simulink model "EPS_sim_test_v5_R19a"  (R2018b)
settings: Solver=FixedStepAuto  StartTime=0.0  StopTime=tsimulation  FixedStep=delta_t  MaxStep=10  RelTol=1e-3
values from neighbouring files (symbols this model uses):
  C = Cbat*Nbp*3600    (= 37440)    [demoEPS.m]    (also in demoEPS_R2019a.m; demoEPS_v1.m; demoEPS_v1a.m; demoEPS_v1test.m)
  DOD_0 = 0    [demoEPS.m]    (also in demoEPS_R2019a.m; demoEPS_v1.m; demoEPS_v1a.m; demoEPS_v1test.m)
  eff_ADC1 = 0.6    [demoEPS_v5.m]
  eff_GPS = 0.94    [demoEPS_v5.m]
  eff_MTQ = 0.91    [demoEPS_v5.m]
  eff_OBC = 0.95    [demoEPS_v4.m]    (also in demoEPS_v5.m = 0.94)
  eff_RWA = 0.3    [demoEPS_v5.m]
  eff_S = 0.98    [demoEPS_v5.m]
  eff_UHF = 0.94    [demoEPS_v5.m]
  EN_ADCS1 = 1    [demoEPS_v5.m]
  EN_GPS = 1    [demoEPS_v5.m]
  EN_heat = 0    [demoEPS_v5.m]
  EN_MTQ = 1    [demoEPS_v5.m]
  EN_OBC = 1    [demoEPS_v5.m]
  EN_RWA = 1    [demoEPS_v5.m]
  EN_S = 1    [demoEPS_v5.m]
  EN_UHF = 1    [demoEPS_v5.m]
  I_BC_max = -input (4)    [battchargedischarge.m]    (also in demoEPS.m = 3; demoEPS_R2019a.m = 3; demoEPS_v1.m = 3; demoEPS_v1a.m = 3)
  I_BD_max = input (3)    [battchargedischarge.m]    (also in demoEPS.m = 5; demoEPS_R2019a.m = 5; demoEPS_v1.m = 5; demoEPS_v1a.m = 5)
  Nbs = math.ceil(Vbusmin/Vbatmin)    [calc_mass_EPS.m]    (also in demoEPS.m = 4; demoEPS_R2019a.m = 4; demoEPS_v1.m = 4; demoEPS_v1a.m = 4)
  P_ADC = 0.55    [demoEPS_v5.m]
  P_eps = 0.6    [demoEPS.m]    (also in demoEPS_R2019a.m; demoEPS_v1.m; demoEPS_v1a.m; demoEPS_v1test.m)
  P_GPS = 0.225    [demoEPS_v5.m]
  P_heater = 3    [demoEPS_v4.m]    (also in demoEPS_v5.m = 6)
  P_MTQ = 1.2    [demoEPS_v5.m]
  P_OBC = 2.15    [demoEPS_v5.m]
  P_RWA = 0.6    [demoEPS_v5.m]
  Psa = 48    [demoEPS.m]    (also in demoEPS_R2019a.m; demoEPS_v1.m; demoEPS_v1a.m; demoEPS_v1test.m)
  Torb = 2*pi*sqrt(a^3/(3.986004418E5))    [demoEPS_v4.m]    (also in demoEPS_v5.m)
libraries: simulink x3
settings Model: Creator=Ricardo  LastModifiedBy=colpari
settings DataIOCC: ReturnWorkspaceOutputs=on

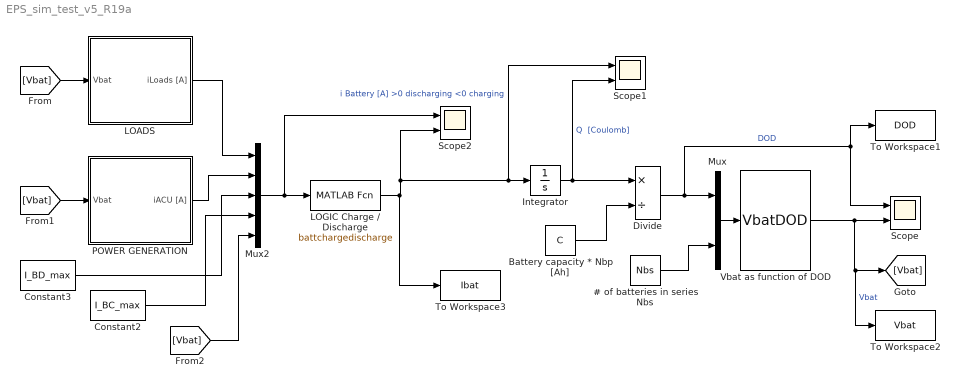
== system EPS_sim_test_v5_R19a ==
  # of batteries in series Nbs : Constant  Value=Nbs
  Battery capacity * Nbp [Ah] : Constant  Value=C
  Constant2 : Constant  Value=I_BC_max
  Constant3 : Constant  Value=I_BD_max
  Divide : Product  Inputs=*/
  Integrator : Integrator  InitialCondition=DOD_0
  LOADS : Subsystem
  LOGIC Charge / Discharge : MATLABFcn  MATLABFcn=battchargedischarge
  Mux : Mux  Inputs=2
  Mux2 : Mux  Inputs=5
  POWER GENERATION : Subsystem
  Scope : Scope  NumInputPorts=2
  Scope1 : Scope  NumInputPorts=2
  Scope2 : Scope  NumInputPorts=2
  To Workspace1 : ToWorkspace  VariableName=DOD  SaveFormat=Timeseries  SampleTime=-1
  To Workspace2 : ToWorkspace  VariableName=Vbat  SaveFormat=Timeseries  SampleTime=-1
  To Workspace3 : ToWorkspace  VariableName=Ibat  SaveFormat=Timeseries  SampleTime=-1
  Vbat as function of DOD : MATLABFcn  MATLABFcn=VbatDOD
  wires:
  Mux/1 -> Vbat as function of DOD/1
  # of batteries in series Nbs/1 -> Mux/2
  Vbat as function of DOD/1 -> To Workspace2/1, [Vbat], Scope/2  "Vbat"
  Divide/1 -> To Workspace1/1, Scope/1, Mux/1  "DOD"
  Integrator/1 -> Scope1/2, Divide/1  "Q  [Coulomb]"
  Battery capacity * Nbp [Ah]/1 -> Divide/2
  [Vbat] -> LOADS/1(Vbat)
  POWER GENERATION/1(iACU [A]) -> Mux2/2
  [Vbat] -> POWER GENERATION/1(Vbat)
  LOADS/1(iLoads [A]) -> Mux2/1
  Mux2/1 -> LOGIC Charge / Discharge/1, Scope2/1
  Constant3/1 -> Mux2/3
  Constant2/1 -> Mux2/4
  LOGIC Charge / Discharge/1 -> To Workspace3/1, Scope1/1, Integrator/1, Scope2/2  "i Battery [A] >0 discharging <0 charging"
  [Vbat] -> Mux2/5

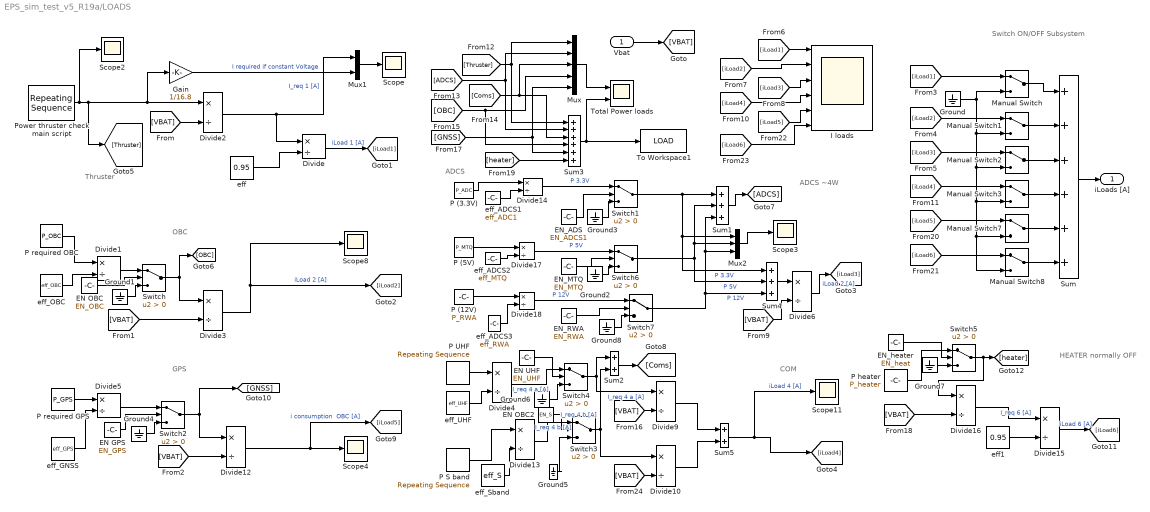
== system EPS_sim_test_v5_R19a/LOADS ==
  note: Switch
      | ON/OFF
      | Subsystem
  note: ADCS
  note: Thruster
  note: OBC
  note: ADCS ~4W
  note: COM
  note: GPS
  note: HEATER
      | normally
      | OFF
  Vbat : Inport
  Divide{,1..6,9..10,12..18} (16 alike) : Product  Inputs=*/
  EN GPS : Constant  Value=EN_GPS
  EN OBC : Constant  Value=EN_OBC
  EN OBC2 : Constant  Value=EN_S
  EN UHF : Constant  Value=EN_UHF
  EN_ADS : Constant  Value=EN_ADCS1
  EN_MTQ : Constant  Value=EN_MTQ
  EN_RWA : Constant  Value=EN_RWA
  EN_heater : Constant  Value=EN_heat
  Gain : Gain  Gain=1/16.8
  Ground{,1..8} (9 alike) : Ground
  I loads : Scope  NumInputPorts=6
  Manual Switch{,1..3,7..8} (6 alike) : ManualSwitch
  Mux : Mux  Inputs=5
  Mux1 : Mux  Inputs=2
  Mux2 : Mux  Inputs=3
  P (12V) : Constant  Value=P_RWA
  P (3.3V) : Constant  Value=P_ADC
  P (5V) : Constant  Value=P_MTQ
  "P S band " : simulink/Sources/Repeating Sequence  rep_seq_t=t_tx_S  rep_seq_y=p_tx_S
  "P UHF " : simulink/Sources/Repeating Sequence  rep_seq_t=t_tx_UHF  rep_seq_y=p_tx_UHF
  P heater : Constant  Value=P_heater
  P required GPS : Constant  Value=P_GPS
  P required OBC : Constant  Value=P_OBC
  Power thruster check main script : simulink/Sources/Repeating Sequence  rep_seq_t=t_thr  rep_seq_y=p_thr
  Scope{,2..4,8,11} (6 alike) : Scope
  Sum : Sum  Inputs=++++++
  Sum1 : Sum  Inputs=+++
  Sum2 : Sum
  Sum3 : Sum  Inputs=++++++
  Sum4 : Sum  Inputs=+++
  Sum5 : Sum
  Switch{,1..7} (8 alike) : Switch  Criteria=u2 > Threshold
  To Workspace1 : ToWorkspace  VariableName=LOAD  SaveFormat=Timeseries  SampleTime=-1
  Total Power loads : Scope  NumInputPorts=2
  eff : Constant  Value=0.95
  eff1 : Constant  Value=0.95
  "eff_ADCS1 " : Constant  Value=eff_ADC1
  eff_ADCS2 : Constant  Value=eff_MTQ
  "eff_ADCS3 " : Constant  Value=eff_RWA
  eff_GNSS : Constant  Value=eff_GPS
  eff_OBC : Constant  Value=eff_OBC
  eff_Sband : Constant  Value=eff_S
  eff_UHF : Constant  Value=eff_UHF
  iLoads [A] : Outport
  wires:
  Gain/1 -> Mux1/2  "I required if constant Voltage"
  Divide2/1 -> Divide/1, Mux1/1  "I_req 1 [A]"
  [VBAT] -> Divide3/2
  Vbat/1 -> [VBAT]
  [VBAT] -> Divide2/2
  Sum/1 -> iLoads [A]/1
  Mux1/1 -> Scope/1
  eff_OBC/1 -> Divide1/2
  Power thruster check main script/1 -> Scope2/1, [Thruster], Gain/1, Divide2/1
  eff/1 -> Divide/2
  Divide/1 -> [iLoad1]  "iLoad 1 [A]"
  Manual Switch/1 -> Sum/1
  Manual Switch1/1 -> Sum/2
  Manual Switch2/1 -> Sum/3
  [iLoad2] -> I loads/2
  [iLoad1] -> I loads/1
  [iLoad3] -> I loads/3
  Sum1/1 -> [ADCS]
  P (3.3V)/1 -> Divide14/1
  Sum5/1 -> Scope11/1, [iLoad4]  "iLoad 4 [A]"
  [iLoad4] -> I loads/4
  Manual Switch3/1 -> Sum/4
  "P UHF "/1 -> Divide4/1
  [iLoad4] -> Manual Switch3/1
  [iLoad3] -> Manual Switch2/1
  [iLoad2] -> Manual Switch1/1
  [iLoad1] -> Manual Switch/1
  Ground/1 -> Manual Switch/2, Manual Switch8/2, Manual Switch7/2, Manual Switch3/2, Manual Switch2/2, Manual Switch1/2
  Mux/1 -> Total Power loads/1
  [Thruster] -> Sum3/1, Mux/1
  [ADCS] -> Sum3/2, Mux/2
  [Coms] -> Sum3/3, Mux/3
  [OBC] -> Sum3/4, Mux/4
  [heater] -> Sum3/6
  Sum3/1 -> Total Power loads/2, To Workspace1/1
  Divide12/1 -> [iLoad5], Scope4/1  "i consumption  OBC [A]"
  [VBAT] -> Divide12/2
  eff_GNSS/1 -> Divide5/2
  [GNSS] -> Sum3/5, Mux/5
  eff1/1 -> Divide15/2
  Divide15/1 -> [iLoad6]  "iLoad 6 [A]"
  P heater/1 -> Switch5/1
  Divide16/1 -> Divide15/1  "I_req 6 [A]"
  [VBAT] -> Divide16/2
  Switch5/1 -> Divide16/1, [heater]
  Manual Switch7/1 -> Sum/5
  Manual Switch8/1 -> Sum/6
  [iLoad6] -> Manual Switch8/1
  [iLoad5] -> Manual Switch7/1
  [iLoad5] -> I loads/5
  [iLoad6] -> I loads/6
  P (5V)/1 -> Divide17/1
  P (12V)/1 -> Divide18/1
  "eff_ADCS1 "/1 -> Divide14/2
  "eff_ADCS3 "/1 -> Divide18/2
  eff_ADCS2/1 -> Divide17/2
  Switch1/1 -> Mux2/1, Sum4/1, Sum1/1  "P 3.3V"
  Switch6/1 -> Sum4/2, Sum1/2, Mux2/2  "P 5V"
  Switch7/1 -> Sum1/3, Mux2/3, Sum4/3  "P 12V"
  Sum4/1 -> Divide6/1
  P required OBC/1 -> Divide1/1
  Switch/1 -> Divide3/1, [OBC]
  Divide3/1 -> Scope8/1, [iLoad2]  "iLoad 2 [A]"
  P required GPS/1 -> Divide5/1
  Switch2/1 -> [GNSS], Divide12/1
  "P S band "/1 -> Divide13/1
  eff_Sband/1 -> Divide13/2
  Switch4/1 -> Divide9/1, Sum2/1  "I_req 4 a [A]"
  Switch3/1 -> Sum2/2, Divide10/1  "I_req 4 b [A]"
  Sum2/1 -> [Coms]
  eff_UHF/1 -> Divide4/2
  [VBAT] -> Divide9/2
  [VBAT] -> Divide10/2
  Divide10/1 -> Sum5/2
  Divide9/1 -> Sum5/1
  [VBAT] -> Divide6/2
  Divide6/1 -> [iLoad3]  "iLoad 2 [A]"
  Divide1/1 -> Switch/1
  EN OBC/1 -> Switch/2
  Ground1/1 -> Switch/3
  Ground4/1 -> Switch2/3
  EN GPS/1 -> Switch2/2
  Divide5/1 -> Switch2/1
  Ground5/1 -> Switch3/3
  EN OBC2/1 -> Switch3/2
  EN UHF/1 -> Switch4/2
  Ground6/1 -> Switch4/3
  Divide4/1 -> Switch4/1  "I_req 4 a [A]"
  Divide13/1 -> Switch3/1  "I_req 4 b [A]"
  Ground7/1 -> Switch5/3
  EN_heater/1 -> Switch5/2
  Mux2/1 -> Scope3/1
  Ground3/1 -> Switch1/3
  EN_ADS/1 -> Switch1/2
  Ground2/1 -> Switch6/3
  EN_MTQ/1 -> Switch6/2
  Ground8/1 -> Switch7/3
  EN_RWA/1 -> Switch7/2
  Divide18/1 -> Switch7/1  "P 12V"
  Divide14/1 -> Switch1/1  "P 3.3V"
  Divide17/1 -> Switch6/1  "P 5V"

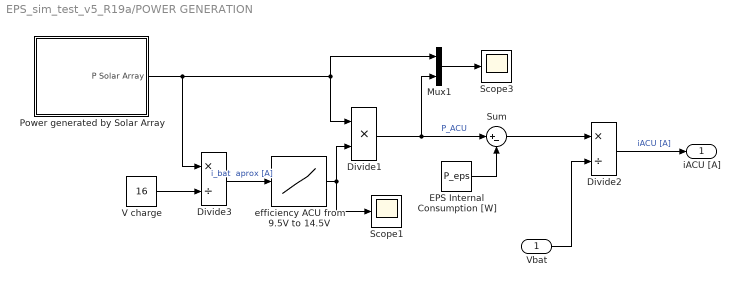
== system EPS_sim_test_v5_R19a/POWER GENERATION ==
  Vbat : Inport
  Divide1 : Product  Inputs=**
  Divide2 : Product  Inputs=*/
  Divide3 : Product  Inputs=*/
  EPS Internal Consumption [W] : Constant  Value=P_eps
  Mux1 : Mux  Inputs=2
  Power generated by Solar Array : Subsystem
  Scope1 : Scope
  Scope3 : Scope
  Sum : Sum  Inputs=|+-
  V charge : Constant  Value=16
  efficiency ACU from 9.5V to 14.5V : Lookup_n-D  NumberOfTableDimensions=1  BreakpointsForDimension1=[0,0.13,0.16,0.236,0.4187,0.654,0.684,0.745,0.801,0.9372,1.046,1.16,1.21,1.5,1.66,2,4]  Table=[0.905,0.928,0.9296,0.9296,0.9337,0.9296,0.9296,0.9296,0.9275,0.9275,0.9254,0.9254,0.9234,0.9193,0.9193,0.9134,0.9134]  InternalRulePriority=Speed  RndMeth=Simplest  InputSameDT=on
  iACU [A] : Outport
  wires:
  Divide2/1 -> iACU [A]/1  "iACU [A]"
  Mux1/1 -> Scope3/1
  Vbat/1 -> Divide2/2
  efficiency ACU from 9.5V to 14.5V/1 -> Scope1/1, Divide1/2
  Divide1/1 -> Sum/1, Mux1/2  "P_ACU"
  Sum/1 -> Divide2/1
  EPS Internal Consumption [W]/1 -> Sum/2
  Divide3/1 -> efficiency ACU from 9.5V to 14.5V/1  "i_bat  aprox [A]"
  V charge/1 -> Divide3/2
  Power generated by Solar Array/1(P Solar Array) -> Divide3/1, Divide1/1, Mux1/1

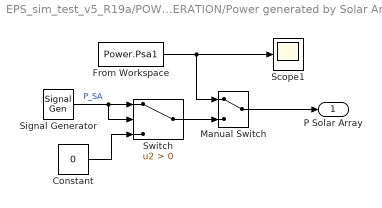
== system EPS_sim_test_v5_R19a/POWER GENERATION/Power generated by Solar Array ==
  Constant : Constant  Value=0
  From Workspace : FromWorkspace  VariableName=Power.Psa1
  Manual Switch : ManualSwitch
  Scope1 : Scope
  Signal Generator : SignalGenerator  Amplitude=-Psa  Frequency=1/Torb
  Switch : Switch  Criteria=u2 > Threshold
  P Solar Array : Outport
  wires:
  From Workspace/1 -> Manual Switch/1, Scope1/1
  Constant/1 -> Switch/3
  Signal Generator/1 -> Switch/2, Switch/1  "P_SA"
  Manual Switch/1 -> P Solar Array/1
  Switch/1 -> Manual Switch/2
